simulink model "work2"  (R2024b)
settings: Solver=VariableStepAuto  StartTime=0.0  StopTime=0.3  FixedStep=1e-6  RelTol=1e-5
values from neighbouring files (symbols this model uses):
  C1 = 4700e-6    (= 0.0047)    [variables.m]
  C2 = 3300e-6    (= 0.0033)    [variables.m]
  D = Uo / (Us + Uo)    (= 0.555555555556)    [variables.m]
  L1 = 2.6e-5    (= 2.6e-05)    [variables.m]
  L2 = 1.04e-4    (= 0.000104)    [variables.m]
  R = 5    [variables.m]
  Ts = 1  / fs    (= 1e-05)    [variables.m]
  Us = 20    [variables.m]
libraries: spsVoltageMeasurementLib x7, spsSeriesRLCBranchLib x5, spsCurrentMeasurementLib x5, spsDiodeLib x1, spsMosfetLib x1, spsDCVoltageSourceLib x1, sps_lib x1
settings Model: Creator=86195  LastModifiedBy=86195

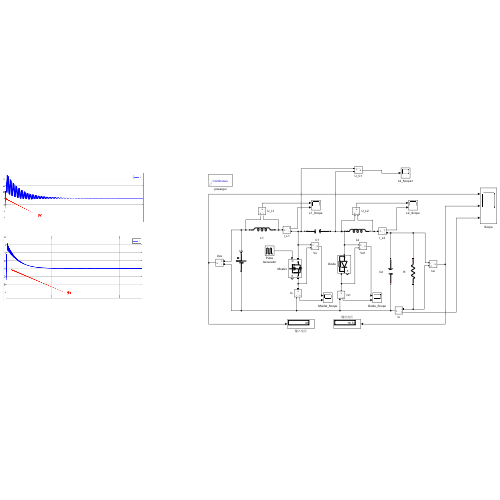
[thumbnail: Simulink's stored preview of the top-level diagram]
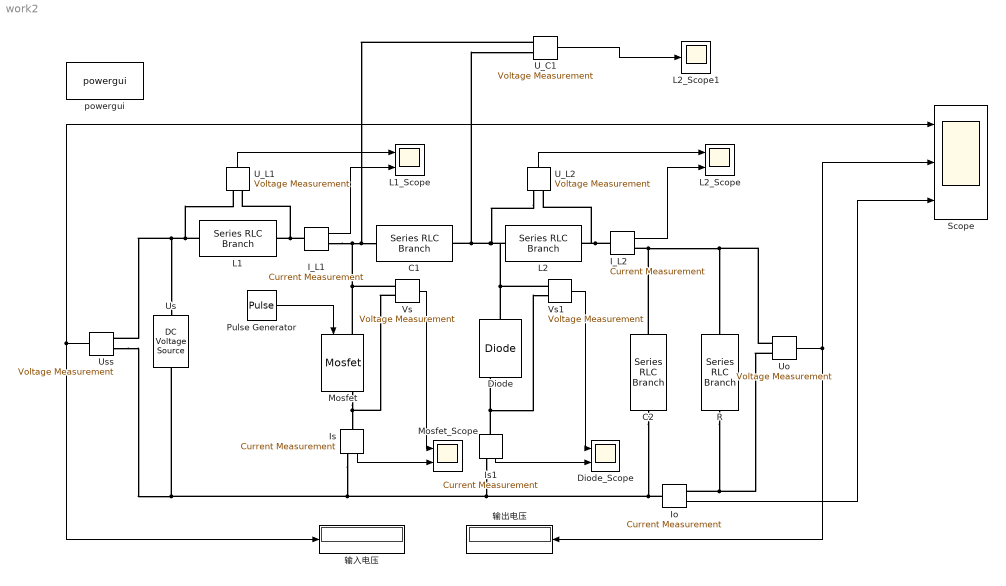
== system work2 ==
  C1 : spsSeriesRLCBranchLib/Series RLC Branch  LConnTagsString=__new0  RConnTagsString=__new0  BranchType=C  Resistance=1  Inductance=1e-3  SetiL0=off  InitialCurrent=0  Capacitance=C1  Setx0=off  InitialVoltage=0  Measurements=None
  C2 : spsSeriesRLCBranchLib/Series RLC Branch  LConnTagsString=__new0  RConnTagsString=__new0  BranchType=C  Resistance=1  Inductance=1e-3  SetiL0=off  InitialCurrent=0  Capacitance=C2  Setx0=off  InitialVoltage=0  Measurements=None
  Diode : spsDiodeLib/Diode  Ron=0.001  Lon=0  Vf=0.0  IC=0  UseSnubber=0  Rs=500  Cs=250e-9  Measurements=on
  Diode_Scope : Scope  NumInputPorts=2
  I_L1 : spsCurrentMeasurementLib/Current Measurement  PhasorSimulation=off  OutputType=Complex  PSBequivalent=0
  I_L2 : spsCurrentMeasurementLib/Current Measurement  PhasorSimulation=off  OutputType=Complex  PSBequivalent=0
  Io : spsCurrentMeasurementLib/Current Measurement  PhasorSimulation=off  OutputType=Complex  PSBequivalent=0
  Is : spsCurrentMeasurementLib/Current Measurement  PhasorSimulation=off  OutputType=Complex  PSBequivalent=0
  Is1 : spsCurrentMeasurementLib/Current Measurement  PhasorSimulation=off  OutputType=Complex  PSBequivalent=0
  L1 : spsSeriesRLCBranchLib/Series RLC Branch  LConnTagsString=__new0  RConnTagsString=__new0  BranchType=L  Resistance=1  Inductance=L1  SetiL0=off  InitialCurrent=0  Capacitance=1e-6  Setx0=off  InitialVoltage=0  Measurements=None
  L1_Scope : Scope  NumInputPorts=2
  L2 : spsSeriesRLCBranchLib/Series RLC Branch  LConnTagsString=__new0  RConnTagsString=__new0  BranchType=L  Resistance=1  Inductance=L2  SetiL0=off  InitialCurrent=0  Capacitance=1e-6  Setx0=off  InitialVoltage=0  Measurements=None
  L2_Scope : Scope  NumInputPorts=2
  L2_Scope1 : Scope
  Mosfet : spsMosfetLib/Mosfet  Ron=0.00001  Lon=0  Rd=0.01  Vfd=0  IC=0  Rs=1e5  Cs=inf  Measurements=on
  Mosfet_Scope : Scope  NumInputPorts=2
  Pulse Generator : DiscretePulseGenerator  PulseType=Time based  Period=Ts  PulseWidth=D*100
  R : spsSeriesRLCBranchLib/Series RLC Branch  LConnTagsString=__new0  RConnTagsString=__new0  BranchType=R  Resistance=R  Inductance=1e-3  SetiL0=off  InitialCurrent=0  Capacitance=1e-6  Setx0=off  InitialVoltage=0  Measurements=None
  Scope : Scope  NumInputPorts=3
  U_C1 : spsVoltageMeasurementLib/Voltage Measurement  PhasorSimulation=off  OutputType=Complex  PSBequivalent=0
  U_L1 : spsVoltageMeasurementLib/Voltage Measurement  PhasorSimulation=off  OutputType=Complex  PSBequivalent=0
  U_L2 : spsVoltageMeasurementLib/Voltage Measurement  PhasorSimulation=off  OutputType=Complex  PSBequivalent=0
  Uo : spsVoltageMeasurementLib/Voltage Measurement  PhasorSimulation=off  OutputType=Complex  PSBequivalent=0
  Us : spsDCVoltageSourceLib/DC Voltage Source  Amplitude=Us  Measurements=None
  Uss : spsVoltageMeasurementLib/Voltage Measurement  PhasorSimulation=off  OutputType=Complex  PSBequivalent=0
  Vs : spsVoltageMeasurementLib/Voltage Measurement  PhasorSimulation=off  OutputType=Complex  PSBequivalent=0
  Vs1 : spsVoltageMeasurementLib/Voltage Measurement  PhasorSimulation=off  OutputType=Complex  PSBequivalent=0
  powergui : sps_lib/powergui  Priority=1  SimulationMode=Continuous  SampleTime=50e-6  frequency=60  Iterations=50  frequencyindice=0  Pbase=100e6  ErrMax=1e-4  UnitsV=kV  UnitsW=MW  buscounter=0  FunctionMessages=off  echomessages=off  EnableUseOfTLC=off  CurrentSourceSwitches=off  DisableSnubberDevices=off  DisableRonSwitches=off  DisableVfSwitches=off  DisplayEquations=off  AutomaticDiscreteSolvers=off  SolverType=Tustin/Backward Euler (TBE)  Interpol=off  ExternalGateDelay=off  methode=off  Ts=100  x0status=blocks  SPID=on  SwTol=0  HookPort=off  NonlinearTolerance=1e-4  nMaxIteration=100  ContinueOnMaxIteration=off  RestoreLinks=warning  ResistiveCurrentMeasurement=off  Frange=[0:2:500]  Ylog=off  Xlog=on  ShowGrid=off  save=off  variable=ZData  structure=0  ZoomFFT=off  StartTime=0.0  cycles=1  DisplayStyle=1  fundamental=60  FreqAxis=off  MaxFrequency=1000  frequencyindicesteady=1  RmsSteady=1  display=off
  输入电压 : Display
  输出电压 : Display
  wires:
  Uo/1 -> Scope/2, 输出电压/1
  Uss/1 -> 输入电压/1, Scope/1
  Io/1 -> Scope/3
  U_L2/1 -> L2_Scope/1
  I_L2/1 -> L2_Scope/2
  U_L1/1 -> L1_Scope/1
  I_L1/1 -> L1_Scope/2
  Vs/1 -> Mosfet_Scope/1
  Is/1 -> Mosfet_Scope/2
  Is1/1 -> Diode_Scope/2
  Vs1/1 -> Diode_Scope/1
  Pulse Generator/1 -> Mosfet/1
  U_C1/1 -> L2_Scope1/1
  connections:
  Mosfet/LConn1 -- Vs/LConn1 -- I_L1/RConn1 -- U_C1/LConn1 -- C1/LConn1
  L2/LConn1 -- Diode/LConn1 -- Vs1/LConn1 -- U_L2/LConn1 -- U_C1/LConn2 -- C1/RConn1
  C2/RConn1 -- I_L2/RConn1 -- Uo/LConn2 -- R/LConn1
  C2/LConn1 -- Uss/LConn2 -- Us/LConn1 -- Is/RConn1 -- Is1/RConn1 -- Io/LConn1
  R/RConn1 -- Uo/LConn1 -- Io/RConn1
  L1/LConn1 -- U_L1/LConn1 -- Us/RConn1 -- Uss/LConn1
  I_L2/LConn1 -- U_L2/LConn2 -- L2/RConn1
  I_L1/LConn1 -- U_L1/LConn2 -- L1/RConn1
  Vs/LConn2 -- Is/LConn1 -- Mosfet/RConn1
  Is1/LConn1 -- Vs1/LConn2 -- Diode/RConn1
